simulink model "TeslaCoil"  (R2024a)
settings: Solver=VariableStepAuto  StartTime=0.0  StopTime=10.0  RelTol=1e-3
undefined symbols (not defined in the file): DiscIntNeverNeededParam
libraries: nesl_utility x4, simulink x1
settings Model: Creator=Perij  LastModifiedBy=Perij

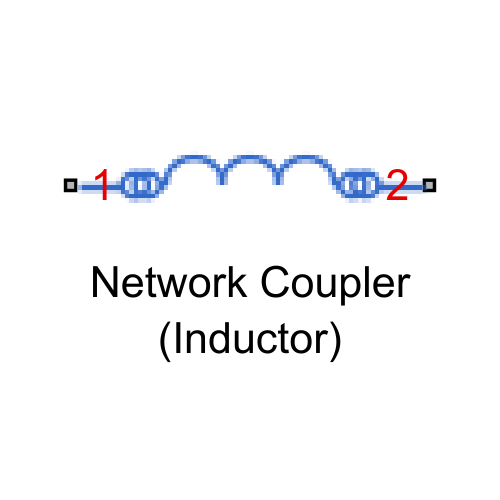
[thumbnail: Simulink's stored preview of the top-level diagram]
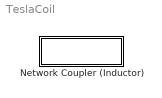
== system TeslaCoil ==
  Network Coupler (Inductor) : Subsystem  mask(Network Coupler (Inductor)){}
      mask init:
      | % Icon
      | key = 'Simscape.NetworkCouplers.Inductor';
      | foundation.internal.couplers.updateIcon(gcb,'inductor.svg',key)
      settings: OpenFcn=open_system(gcbh,'force')
      mask Help: web([docroot '/simscape/ref/networkcouplerinductor.html'])
      mask Display:
      | color('red');
      | port_label('LConn', 1,'1')
      | port_label('RConn', 1,'2')

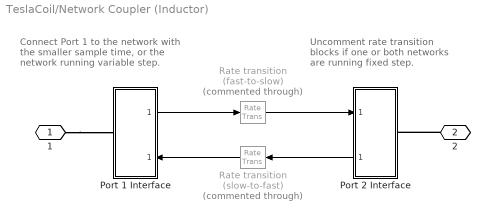
== system TeslaCoil/Network Coupler (Inductor) ==
  note: Connect Port 1 to the network
      | with the smaller sample time, or
      | the network running variable step.
  note: Uncomment rate transition
      | blocks if one or both networks
      | are running fixed step.
  Port 1 Interface : Subsystem  mask(Network Coupler (Inductor) Port 1 Interface){isThreePhase=off, numNodes=1, inductance=1e-3, samplingType=Variable step at ports 1 and 2, h1=0.0002, h2=0.001, predictionDiscreteToContinuous=off, smoothingContinuousToDiscrete=off, predictionSlowToFast=off, smoothingFastToSlow=off, nSmooth=1, tsSmoothing=0.01, rNetwork=0.1, hRecommended=0.001, i0=0}
      mask prompts: isThreePhase "physmod:simscape:couplers:SimscapeNetworkCouplersLib:ElectricalThreePhase_MP"; numNodes "physmod:simscape:couplers:SimscapeNetworkCouplersLib:ElectricalNodeArraySize_MP"; inductance "physmod:simscape:couplers:SimscapeNetworkCouplersLib:InductanceH_MP"; samplingType "physmod:simscape:couplers:SimscapeNetworkCouplersLib:SamplingType_MP"; h1 "physmod:simscape:couplers:SimscapeNetworkCouplersLib:Port1NetworkDiscreteSampleTimes_MP"; h2 "physmod:simscape:couplers:SimscapeNetworkCouplersLib:Port2NetworkDiscreteSampleTimes_MP"; predictionDiscreteToContinuous "physmod:simscape:couplers:SimscapeNetworkCouplersLib:UsePredictionWhenConnectingFixedStepToVariableStep_MP"; smoothingContinuousToDiscrete "physmod:simscape:couplers:SimscapeNetworkCouplersLib:UseSmoothingWhenConnectingVariableStepToFixedStep_MP"; predictionSlowToFast "physmod:simscape:couplers:SimscapeNetworkCouplersLib:UsePredictionWhenConnectingSlowToFastSampleTimes_MP"; smoothingFastToSlow "physmod:simscape:couplers:SimscapeNetworkCouplersLib:UseSmoothingWhenConnectingFastToSlowSampleTimes_MP"; nSmooth "physmod:simscape:couplers:SimscapeNetworkCouplersLib:NumberOfSamplesOverWhichToSmooth_MP"; tsSmoothing "physmod:simscape:couplers:SimscapeNetworkCouplersLib:SmoothingTimeConstants_MP"; rNetwork "physmod:simscape:couplers:SimscapeNetworkCouplersLib:ApproximateConnectedNetworkImpedanceohms_MP"; hRecommended "physmod:simscape:couplers:SimscapeNetworkCouplersLib:RecommendedMaxDiscreteSampleTimes_MP"; i0 "physmod:simscape:couplers:SimscapeNetworkCouplersLib:InitialCurrentA_MP"
      mask help: physmod:simscape:couplers:SimscapeNetworkCouplersLib:NetworkCouplerInductorPort1Interface_MD
      mask init:
      | % Fixed step sample time value check
      | foundation.internal.couplers.checkSampleTimes(gcb,h1,h2);
      | 
      | % Remaining parameter value checks
      | foundation.internal.couplers.electrical.checkParametersInductor(inductance,isThreePhase,numNodes,i0);
      settings: PortSchema="{\"entries\":[{\"content\":{\"sides\":[{\"content\":{\"connectorIds\":[\"LConn1\"]},\"type\":\"ConnectorPlacement.EquallySpacedRectSide\",\"uuid\":\"a6d4a9fd-b5aa-40dc-ab7e-2b646b9b57bc\"},{\"content\":{\"connectorIds\":[\"Out1\",\"In1\"],\"side\":\"RIGHT\"},\"type\":\"ConnectorPlacement.EquallySpacedRectSide\",\"uuid\":\"31bb6273-5b9b-48d0-a1a2-6fbacb979b97\"},{\"content\":{\"connectorIds\":[],\"side\":\"TOP\"},\"type\":\"ConnectorPlacement.EquallySpacedRectSide\",\"uuid\":\"0f7afab2-4481-486c-9ad0-2b42c5b091a4\"}]},\"type\":\"ConnectorPlacement.EquallySpacedConnector\",\"uuid\":\"a98e47aa-cbfd-441a-b14c-c9ea515c056e\"}],\"packageUris\":[\"http://schema.mathworks.com/mf0/Connector/R2020b\"],\"version\":\"1.0\"}"
      mask Help: web([docroot '/simscape/ref/networkcouplerinductor.html'])
      mask Callback isThreePhase: foundation.internal.couplers.electrical.parameterVisibilitiesThreePhase(gcb)
      mask TypeOptions samplingType: physmod:simscape:couplers:SimscapeNetworkCouplersLib:VariableStepAtPorts1And2_PV | physmod:simscape:couplers:SimscapeNetworkCouplersLib:VariableStepAtPort1AndFixedStepAtPort2_PV | physmod:simscape:couplers:SimscapeNetworkCouplersLib:FixedStepBothPortsWithCommonSampleTime_PV | physmod:simscape:couplers:SimscapeNetworkCouplersLib:FixedStepBothPortsWithFasterSamplingAtPort1_PV
      mask Callback samplingType: foundation.internal.couplers.electrical.parameterVisibilities(gcb)
      mask Callback predictionDiscreteToContinuous: foundation.internal.couplers.electrical.parameterVisibilities(gcb)
      mask Callback smoothingContinuousToDiscrete: foundation.internal.couplers.electrical.parameterVisibilities(gcb)
      mask Callback predictionSlowToFast: foundation.internal.couplers.electrical.parameterVisibilities(gcb)
      mask Callback smoothingFastToSlow: foundation.internal.couplers.electrical.parameterVisibilities(gcb)
      mask DialogControl Main Prompt: physmod:simscape:couplers:SimscapeNetworkCouplersLib:tab_Main
      mask DialogControl isThreePhase Prompt: Use three-phase electrical connections
      mask DialogControl numNodes Prompt: Electrical node array size
      mask DialogControl inductance Prompt: Inductance (H)
      mask DialogControl samplingType Prompt: Sampling type
      mask DialogControl h1 Prompt: Port 1 network discrete sample time (s)
      mask DialogControl h2 Prompt: Port 2 network discrete sample time (s)
      mask DialogControl predictionDiscreteToContinuous Prompt: Use prediction when connecting fixed step to variable step
      mask DialogControl smoothingContinuousToDiscrete Prompt: Use smoothing when connecting variable step to fixed step
      mask DialogControl predictionSlowToFast Prompt: Use prediction when connecting slow to fast sample times
      mask DialogControl smoothingFastToSlow Prompt: Use smoothing when connecting fast to slow sample times
      mask DialogControl nSmooth Prompt: Number of samples over which to smooth
      mask DialogControl tsSmoothing Prompt: Smoothing time constant (s)
      mask DialogControl Analysis Prompt: physmod:simscape:couplers:SimscapeNetworkCouplersLib:tab_Analysis
      mask DialogControl connectedNetworkInfo Prompt: physmod:simscape:couplers:SimscapeNetworkCouplersLib:heading_ConnectedNetworkInformation
      mask DialogControl rNetwork Prompt: Approximate connected network resistance (ohms)
      mask DialogControl derivedValues Prompt: physmod:simscape:couplers:SimscapeNetworkCouplersLib:heading_DerivedValues
      mask DialogControl hRecommended Prompt: Recommended max discrete sample time (s)
      mask DialogControl updateRecommendations Prompt: physmod:simscape:couplers:SimscapeNetworkCouplersLib:button_Update
      mask DialogControl updateRecommendations Callback: foundation.internal.couplers.electrical.analysisInductor(gcb);
      mask DialogControl InitialConditions Prompt: physmod:simscape:couplers:SimscapeNetworkCouplersLib:tab_InitialConditions
      mask DialogControl i0 Prompt: Initial current (A)
  Port 2 Interface : Subsystem  mask(Network Coupler (Inductor) Port 2 Interface){isThreePhase=off, numNodes=1}
      mask prompts: isThreePhase "physmod:simscape:couplers:SimscapeNetworkCouplersLib:ElectricalThreePhase_MP"; numNodes "physmod:simscape:couplers:SimscapeNetworkCouplersLib:ElectricalNodeArraySize_MP"
      mask help: physmod:simscape:couplers:SimscapeNetworkCouplersLib:NetworkCouplerInductorPort2Interface_MD
      mask init:
      | % Parameter value checks
      | foundation.internal.couplers.electrical.checkParametersNumNodes(isThreePhase,numNodes);
      settings: PortSchema="{\"entries\":[{\"content\":{\"sides\":[{\"content\":{\"connectorIds\":[\"In1\",\"Out1\"]},\"type\":\"ConnectorPlacement.EquallySpacedRectSide\",\"uuid\":\"5a4c1550-e77d-42df-bf3e-b81963920de7\"},{\"content\":{\"connectorIds\":[\"RConn1\"],\"side\":\"RIGHT\"},\"type\":\"ConnectorPlacement.EquallySpacedRectSide\",\"uuid\":\"3fd730f7-5937-4563-a365-595aaae9027b\"},{\"content\":{\"connectorIds\":[],\"side\":\"TOP\"},\"type\":\"ConnectorPlacement.EquallySpacedRectSide\",\"uuid\":\"c16e04e4-26e8-4fd6-98d3-59adbef44c0d\"}]},\"type\":\"ConnectorPlacement.EquallySpacedConnector\",\"uuid\":\"5588d8d0-d459-45fe-a303-1ca6654e99d0\"}],\"packageUris\":[\"http://schema.mathworks.com/mf0/Connector/R2020b\"],\"version\":\"1.0\"}"
      mask Help: web([docroot '/simscape/ref/networkcouplerinductor.html'])
      mask Callback isThreePhase: foundation.internal.couplers.electrical.parameterVisibilitiesThreePhase(gcb)
      mask DialogControl isThreePhase Prompt: Use three-phase electrical connections
      mask DialogControl numNodes Prompt: Electrical node array size
  Rate transition (fast-to-slow) : RateTransition  Commented=through  Integrity=off
  Rate transition (slow-to-fast) : RateTransition  Commented=through  Integrity=off
  1 : PMIOPort  Side=Left
  2 : PMIOPort  Port=2  Side=Right
  wires:
  Rate transition (fast-to-slow)/1 -> Port 2 Interface/1(current)
  Rate transition (slow-to-fast)/1 -> Port 1 Interface/1(voltage)
  Port 2 Interface/1(voltage) -> Rate transition (slow-to-fast)/1
  Port 1 Interface/1(current) -> Rate transition (fast-to-slow)/1
  connections:
  1/RConn1 -- Port 1 Interface/LConn1
  2/RConn1 -- Port 2 Interface/RConn1

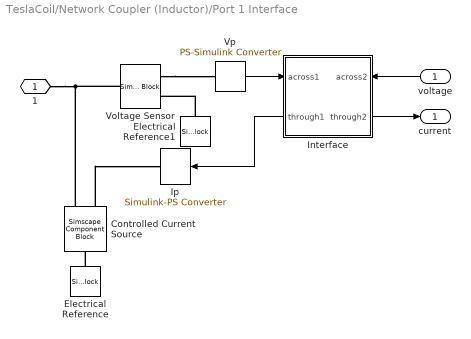
== system TeslaCoil/Network Coupler (Inductor)/Port 1 Interface ==
  voltage : Inport
  Controlled Current Source : SimscapeComponentBlock  SourceFile=foundation.internal.couplers.electrical.currentSource  ComponentPath=foundation.internal.couplers.electrical.currentSource  ComponentVariants="[\"foundation.internal.couplers.electrical.currentSource\"]"  ComponentVariantNames="[\"currentSource\"]"  ClassName=currentSource  SchemaVersion=1  threePhase=false  numNodes=numNodes
      settings: CopyFcn=simscape.engine.sli.internal.componentblockcallback(gcbh,'COPY')  PreCopyFcn=simscape.engine.sli.internal.componentblockcallback(gcbh,'PRECOPY')  PreDeleteFcn=simscape.engine.sli.internal.componentblockcallback(gcbh,'PREDELETE')  InternalSimscapePortConfiguration="{\"Bottom\":[],\"Left\":[{\"id\":\"head\",\"label\":\"\",\"type\":\"foundation.electrical.electrical\"}],\"Right\":[{\"id\":\"iT\",\"label\":\"\",\"type\":\"input\"},{\"id\":\"tail\",\"label\":\"\",\"type\":\"foundation.electrical.electrical\"}],\"Top\":[]}"
      mask Type: Controlled Current Source
  Electrical Reference : SimscapeComponentBlock  SourceFile=foundation.internal.couplers.electrical.reference  ComponentPath=foundation.internal.couplers.electrical.reference  ComponentVariants="[\"foundation.internal.couplers.electrical.reference\"]"  ComponentVariantNames="[\"reference\"]"  ClassName=reference  SchemaVersion=1  threePhase=false  numNodes=numNodes
      settings: CopyFcn=simscape.engine.sli.internal.componentblockcallback(gcbh,'COPY')  PreCopyFcn=simscape.engine.sli.internal.componentblockcallback(gcbh,'PRECOPY')  PreDeleteFcn=simscape.engine.sli.internal.componentblockcallback(gcbh,'PREDELETE')  InternalSimscapePortConfiguration="{\"Bottom\":[],\"Left\":[{\"id\":\"p\",\"label\":\"\",\"type\":\"foundation.electrical.electrical\"}],\"Right\":[],\"Top\":[]}"
      mask Type: Electrical Reference
  Electrical Reference1 : SimscapeComponentBlock  SourceFile=foundation.internal.couplers.electrical.reference  ComponentPath=foundation.internal.couplers.electrical.reference  ComponentVariants="[\"foundation.internal.couplers.electrical.reference\"]"  ComponentVariantNames="[\"reference\"]"  ClassName=reference  SchemaVersion=1  threePhase=false  numNodes=numNodes
      settings: CopyFcn=simscape.engine.sli.internal.componentblockcallback(gcbh,'COPY')  PreCopyFcn=simscape.engine.sli.internal.componentblockcallback(gcbh,'PRECOPY')  PreDeleteFcn=simscape.engine.sli.internal.componentblockcallback(gcbh,'PREDELETE')  InternalSimscapePortConfiguration="{\"Bottom\":[],\"Left\":[{\"id\":\"p\",\"label\":\"\",\"type\":\"foundation.electrical.electrical\"}],\"Right\":[],\"Top\":[]}"
      mask Type: Electrical Reference
  Interface : Subsystem  Variant=on  VariantControlMode=label  VariantControl=Variant1  LabelModeActiveChoice=Continuous
      settings: PortSchema="{\"entries\":[{\"content\":{\"sides\":[{\"content\":{\"connectorIds\":[\"In1\",\"Out2\"]},\"type\":\"ConnectorPlacement.EquallySpacedRectSide\",\"uuid\":\"aa56821c-7799-44e3-b228-553c5b43a68d\"},{\"content\":{\"connectorIds\":[\"In2\",\"Out1\"],\"side\":\"RIGHT\"},\"type\":\"ConnectorPlacement.EquallySpacedRectSide\",\"uuid\":\"8658dee5-55e2-4f33-bdec-e6600ce27fc1\"},{\"content\":{\"connectorIds\":[],\"side\":\"TOP\"},\"type\":\"ConnectorPlacement.EquallySpacedRectSide\",\"uuid\":\"2effe9c6-8e61-4f0c-a39b-329d9ffc707d\"}]},\"type\":\"ConnectorPlacement.EquallySpacedConnector\",\"uuid\":\"c8fc8444-dfc7-49a5-9550-b957635f7d8f\"}],\"packageUris\":[\"http://schema.mathworks.com/mf0/Connector/R2020b\"],\"version\":\"1.0\"}"
  Ip : nesl_utility/Simulink-PS Converter  PhysicalDomain=network_engine_domain  SubClassName=ps_input  LeftPortType=input  RightPortType=output  PseudoPeriodic=off  Frequencies=[]  NoiseDistribution=none  NoiseParameters=[]  Unit=A  AffineConversion=off  FilteringAndDerivatives=zero  SimscapeFilterOrder=1  InputFilterTimeConstant=0.001  UdotUserProvided=1
  Voltage Sensor : SimscapeComponentBlock  SourceFile=foundation.internal.couplers.electrical.voltageSensor  ComponentPath=foundation.internal.couplers.electrical.voltageSensor  ComponentVariants="[\"foundation.internal.couplers.electrical.voltageSensor\"]"  ComponentVariantNames="[\"voltageSensor\"]"  ClassName=voltageSensor  SchemaVersion=1  threePhase=false  numNodes=numNodes
      settings: CopyFcn=simscape.engine.sli.internal.componentblockcallback(gcbh,'COPY')  PreCopyFcn=simscape.engine.sli.internal.componentblockcallback(gcbh,'PRECOPY')  PreDeleteFcn=simscape.engine.sli.internal.componentblockcallback(gcbh,'PREDELETE')  InternalSimscapePortConfiguration="{\"Bottom\":[],\"Left\":[{\"id\":\"p\",\"label\":\"+\",\"type\":\"foundation.electrical.electrical\"}],\"Right\":[{\"id\":\"V\",\"label\":\"V\",\"type\":\"output\"},{\"id\":\"n\",\"label\":\"-\",\"type\":\"foundation.electrical.electrical\"}],\"Top\":[]}"
      mask Type: Voltage Sensor
  Vp : nesl_utility/PS-Simulink Converter  PhysicalDomain=network_engine_domain  SubClassName=ps_output  LeftPortType=input  RightPortType=output  PseudoPeriodic=off  Frequencies=[]  VectorFormat=1-D array  Unit=V  AffineConversion=off
  1 : PMIOPort  Side=Left
  current : Outport
  wires:
  voltage/1 -> Interface/2(across2)
  Interface/2(through1) -> Ip/1
  Vp/1 -> Interface/1(across1)
  Interface/1(through2) -> current/1
  connections:
  Controlled Current Source/RConn1 -- Ip/RConn1
  Electrical Reference/LConn1 -- Controlled Current Source/LConn1
  Electrical Reference1/LConn1 -- Voltage Sensor/RConn2
  Controlled Current Source/RConn2 -- Voltage Sensor/LConn1 -- 1/RConn1
  Voltage Sensor/RConn1 -- Vp/LConn1

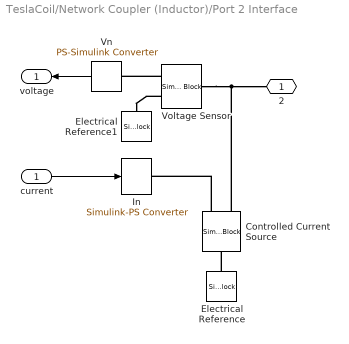
== system TeslaCoil/Network Coupler (Inductor)/Port 2 Interface ==
  current : Inport
  Controlled Current Source : SimscapeComponentBlock  SourceFile=foundation.internal.couplers.electrical.currentSource  ComponentPath=foundation.internal.couplers.electrical.currentSource  ComponentVariants="[\"foundation.internal.couplers.electrical.currentSource\"]"  ComponentVariantNames="[\"currentSource\"]"  ClassName=currentSource  SchemaVersion=1  threePhase=false  numNodes=numNodes
      settings: CopyFcn=simscape.engine.sli.internal.componentblockcallback(gcbh,'COPY')  PreCopyFcn=simscape.engine.sli.internal.componentblockcallback(gcbh,'PRECOPY')  PreDeleteFcn=simscape.engine.sli.internal.componentblockcallback(gcbh,'PREDELETE')  InternalSimscapePortConfiguration="{\"Bottom\":[],\"Left\":[{\"id\":\"head\",\"label\":\"\",\"type\":\"foundation.electrical.electrical\"}],\"Right\":[{\"id\":\"iT\",\"label\":\"\",\"type\":\"input\"},{\"id\":\"tail\",\"label\":\"\",\"type\":\"foundation.electrical.electrical\"}],\"Top\":[]}"
      mask Type: Controlled Current Source
  Electrical Reference : SimscapeComponentBlock  SourceFile=foundation.internal.couplers.electrical.reference  ComponentPath=foundation.internal.couplers.electrical.reference  ComponentVariants="[\"foundation.internal.couplers.electrical.reference\"]"  ComponentVariantNames="[\"reference\"]"  ClassName=reference  SchemaVersion=1  threePhase=false  numNodes=numNodes
      settings: CopyFcn=simscape.engine.sli.internal.componentblockcallback(gcbh,'COPY')  PreCopyFcn=simscape.engine.sli.internal.componentblockcallback(gcbh,'PRECOPY')  PreDeleteFcn=simscape.engine.sli.internal.componentblockcallback(gcbh,'PREDELETE')  InternalSimscapePortConfiguration="{\"Bottom\":[],\"Left\":[{\"id\":\"p\",\"label\":\"\",\"type\":\"foundation.electrical.electrical\"}],\"Right\":[],\"Top\":[]}"
      mask Type: Electrical Reference
  Electrical Reference1 : SimscapeComponentBlock  SourceFile=foundation.internal.couplers.electrical.reference  ComponentPath=foundation.internal.couplers.electrical.reference  ComponentVariants="[\"foundation.internal.couplers.electrical.reference\"]"  ComponentVariantNames="[\"reference\"]"  ClassName=reference  SchemaVersion=1  threePhase=false  numNodes=numNodes
      settings: CopyFcn=simscape.engine.sli.internal.componentblockcallback(gcbh,'COPY')  PreCopyFcn=simscape.engine.sli.internal.componentblockcallback(gcbh,'PRECOPY')  PreDeleteFcn=simscape.engine.sli.internal.componentblockcallback(gcbh,'PREDELETE')  InternalSimscapePortConfiguration="{\"Bottom\":[],\"Left\":[{\"id\":\"p\",\"label\":\"\",\"type\":\"foundation.electrical.electrical\"}],\"Right\":[],\"Top\":[]}"
      mask Type: Electrical Reference
  In : nesl_utility/Simulink-PS Converter  PhysicalDomain=network_engine_domain  SubClassName=ps_input  LeftPortType=input  RightPortType=output  PseudoPeriodic=off  Frequencies=[]  NoiseDistribution=none  NoiseParameters=[]  Unit=A  AffineConversion=off  FilteringAndDerivatives=zero  SimscapeFilterOrder=1  InputFilterTimeConstant=0.001  UdotUserProvided=1
  Vn : nesl_utility/PS-Simulink Converter  PhysicalDomain=network_engine_domain  SubClassName=ps_output  LeftPortType=input  RightPortType=output  PseudoPeriodic=off  Frequencies=[]  VectorFormat=1-D array  Unit=V  AffineConversion=off
  Voltage Sensor : SimscapeComponentBlock  SourceFile=foundation.internal.couplers.electrical.voltageSensor  ComponentPath=foundation.internal.couplers.electrical.voltageSensor  ComponentVariants="[\"foundation.internal.couplers.electrical.voltageSensor\"]"  ComponentVariantNames="[\"voltageSensor\"]"  ClassName=voltageSensor  SchemaVersion=1  threePhase=false  numNodes=numNodes
      settings: CopyFcn=simscape.engine.sli.internal.componentblockcallback(gcbh,'COPY')  PreCopyFcn=simscape.engine.sli.internal.componentblockcallback(gcbh,'PRECOPY')  PreDeleteFcn=simscape.engine.sli.internal.componentblockcallback(gcbh,'PREDELETE')  InternalSimscapePortConfiguration="{\"Bottom\":[],\"Left\":[{\"id\":\"p\",\"label\":\"+\",\"type\":\"foundation.electrical.electrical\"}],\"Right\":[{\"id\":\"V\",\"label\":\"V\",\"type\":\"output\"},{\"id\":\"n\",\"label\":\"-\",\"type\":\"foundation.electrical.electrical\"}],\"Top\":[]}"
      mask Type: Voltage Sensor
  2 : PMIOPort  Side=Right
  voltage : Outport
  wires:
  current/1 -> In/1
  Vn/1 -> voltage/1
  connections:
  Controlled Current Source/RConn1 -- In/RConn1
  Electrical Reference/LConn1 -- Controlled Current Source/LConn1
  Voltage Sensor/RConn2 -- Electrical Reference1/LConn1
  Voltage Sensor/RConn1 -- Vn/LConn1
  Controlled Current Source/RConn2 -- Voltage Sensor/LConn1 -- 2/RConn1

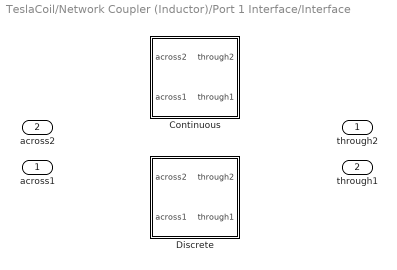
== system TeslaCoil/Network Coupler (Inductor)/Port 1 Interface/Interface ==
  across1 : Inport
  across2 : Inport  Port=2
  Continuous : Subsystem  VariantControl=Continuous
  Discrete : Subsystem  VariantControl=Discrete
  through2 : Outport
  through1 : Outport  Port=2

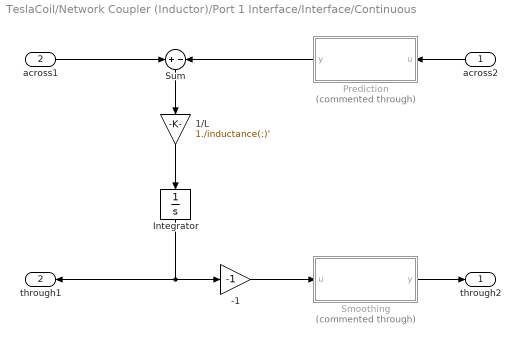
== system TeslaCoil/Network Coupler (Inductor)/Port 1 Interface/Interface/Continuous ==
  across2 : Inport
  across1 : Inport  Port=2
  -1 : Gain  Gain=-1  SaturateOnIntegerOverflow=on  OutDataTypeStr=Inherit: Same as input  ParamDataTypeStr=Inherit: Same as input
  1/L : Gain  Gain=1./inductance(:)'  SaturateOnIntegerOverflow=on  OutDataTypeStr=Inherit: Same as input  ParamDataTypeStr=Inherit: Same as input
  Integrator : Integrator  InitialCondition=i0
  Prediction : Subsystem  Commented=through  mask(Prediction (discrete->continuous)){h2=h2}
      mask prompts: h2 "physmod:simscape:couplers:SimscapeNetworkCouplersLib:PortUDiscreteSampleTimes_MP"
      mask help: physmod:simscape:couplers:SimscapeNetworkCouplersLib:Predictiondiscretecontinuous_MD
      mask DialogControl h2 Prompt: Port u discrete sample time (s)
  Smoothing : Subsystem  Commented=through  mask(Smoothing (continuous->discrete)){tsSmoothing=tsSmoothing, smoothing0=i0}
      mask prompts: tsSmoothing "physmod:simscape:couplers:SimscapeNetworkCouplersLib:SmoothingTimeConstants_MP"; smoothing0 "physmod:simscape:couplers:SimscapeNetworkCouplersLib:InitialOutput_MP"
      mask help: physmod:simscape:couplers:SimscapeNetworkCouplersLib:Smoothingcontinuousdiscrete_MD
      mask DialogControl tsSmoothing Prompt: Smoothing time constant (s)
      mask DialogControl smoothing0 Prompt: Initial output
  Sum : Sum  Inputs=+-  InputSameDT=on  SaturateOnIntegerOverflow=on  OutDataTypeStr=Inherit: Same as first input
  through2 : Outport
  through1 : Outport  Port=2
  wires:
  Integrator/1 -> -1/1, through1/1
  Sum/1 -> 1/L/1
  -1/1 -> Smoothing/1(u)
  1/L/1 -> Integrator/1
  across2/1 -> Prediction/1(u)
  across1/1 -> Sum/1
  Prediction/1(y) -> Sum/2
  Smoothing/1(y) -> through2/1

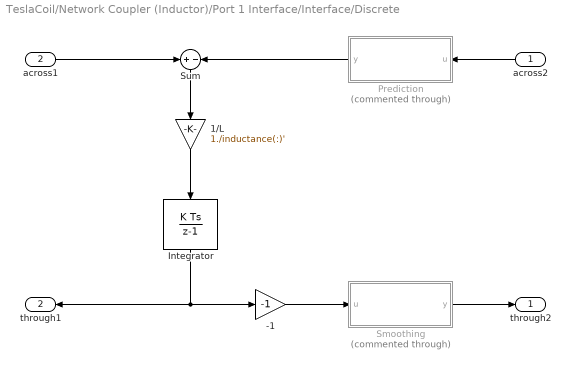
== system TeslaCoil/Network Coupler (Inductor)/Port 1 Interface/Interface/Discrete ==
  across2 : Inport
  across1 : Inport  Port=2
  -1 : Gain  Gain=-1  SaturateOnIntegerOverflow=on  OutDataTypeStr=Inherit: Same as input  ParamDataTypeStr=Inherit: Same as input
  1/L : Gain  Gain=1./inductance(:)'  SaturateOnIntegerOverflow=on  OutDataTypeStr=Inherit: Same as input  ParamDataTypeStr=Inherit: Same as input
  Integrator : DiscreteIntegrator  InitialCondition=i0  SampleTime=h1  ICPrevOutput=DiscIntNeverNeededParam  ICPrevScaledInput=DiscIntNeverNeededParam
  Prediction : Subsystem  Commented=through  mask(Prediction (slow->fast)){h2=h2, h1=h1}
      mask prompts: h2 "physmod:simscape:couplers:SimscapeNetworkCouplersLib:PortUDiscreteSampleTimes_MP"; h1 "physmod:simscape:couplers:SimscapeNetworkCouplersLib:PortYDiscreteSampleTimes_MP"
      mask help: physmod:simscape:couplers:SimscapeNetworkCouplersLib:Predictionslowfast_MD
      mask DialogControl h2 Prompt: Port u discrete sample time (s)
      mask DialogControl h1 Prompt: Port y discrete sample time (s)
  Smoothing : Subsystem  Commented=through  mask(Smoothing (fast->slow)){nSmooth=nSmooth, h1=h1, smoothing0=i0}
      mask prompts: nSmooth "physmod:simscape:couplers:SimscapeNetworkCouplersLib:NumberOfSamplesOverWhichToSmooth_MP"; h1 "physmod:simscape:couplers:SimscapeNetworkCouplersLib:PortUDiscreteSampleTimes_MP"; smoothing0 "physmod:simscape:couplers:SimscapeNetworkCouplersLib:InitialOutput_MP"
      mask help: physmod:simscape:couplers:SimscapeNetworkCouplersLib:Smoothingfastslow_MD
      mask DialogControl nSmooth Prompt: Number of samples over which to smooth
      mask DialogControl h1 Prompt: Port u discrete sample time (s)
      mask DialogControl smoothing0 Prompt: Initial output
  Sum : Sum  Inputs=+-  InputSameDT=on  SaturateOnIntegerOverflow=on  OutDataTypeStr=Inherit: Same as first input
  through2 : Outport
  through1 : Outport  Port=2
  wires:
  Integrator/1 -> -1/1, through1/1
  Sum/1 -> 1/L/1
  -1/1 -> Smoothing/1(u)
  across1/1 -> Sum/1
  across2/1 -> Prediction/1(u)
  1/L/1 -> Integrator/1
  Prediction/1(y) -> Sum/2
  Smoothing/1(y) -> through2/1

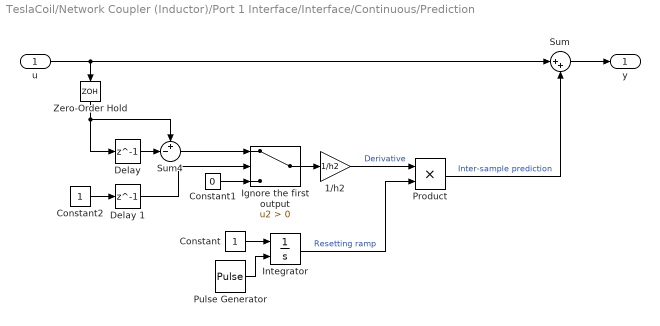
== system TeslaCoil/Network Coupler (Inductor)/Port 1 Interface/Interface/Continuous/Prediction ==
  u : Inport
  1/h2 : Gain  Gain=1/h2
  Constant : Constant  SampleTime=h2
  Constant1 : Constant  Value=0  SampleTime=h2
  Constant2 : Constant  SampleTime=h2
  "Delay " : Delay  DelayLength=1  SampleTime=h2
  Delay 1 : Delay  DelayLength=1  SampleTime=h2
  Ignore the first output : Switch  Criteria=u2 > Threshold  SaturateOnIntegerOverflow=off  InputSameDT=off
  Integrator : Integrator  ExternalReset=either  LimitOutput=on  UpperSaturationLimit=1  LowerSaturationLimit=0
  Product : Product
  Pulse Generator : DiscretePulseGenerator  SampleTime=h2
  Sum : Sum  Inputs=|++
  Sum4 : Sum  Inputs=+-|
  Zero-Order Hold : ZeroOrderHold  SampleTime=h2
  y : Outport
  wires:
  Constant2/1 -> Delay 1/1
  Delay 1/1 -> Ignore the first output/2
  Constant1/1 -> Ignore the first output/3
  Sum4/1 -> Ignore the first output/1
  Ignore the first output/1 -> 1/h2/1
  Pulse Generator/1 -> Integrator/2
  Constant/1 -> Integrator/1
  Integrator/1 -> Product/2  "Resetting ramp"
  Sum/1 -> y/1
  1/h2/1 -> Product/1  "Derivative"
  "Delay "/1 -> Sum4/2
  u/1 -> Zero-Order Hold/1, Sum/1
  Zero-Order Hold/1 -> "Delay "/1, Sum4/1
  Product/1 -> Sum/2  "Inter-sample prediction"

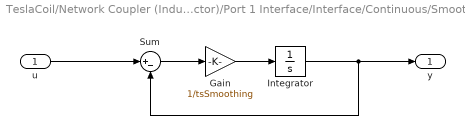
== system TeslaCoil/Network Coupler (Inductor)/Port 1 Interface/Interface/Continuous/Smoothing ==
  u : Inport
  Gain : Gain  Gain=1/tsSmoothing
  Integrator : Integrator  InitialCondition=smoothing0
  Sum : Sum  Inputs=|+-
  y : Outport
  wires:
  Sum/1 -> Gain/1
  Gain/1 -> Integrator/1
  Integrator/1 -> y/1, Sum/2
  u/1 -> Sum/1

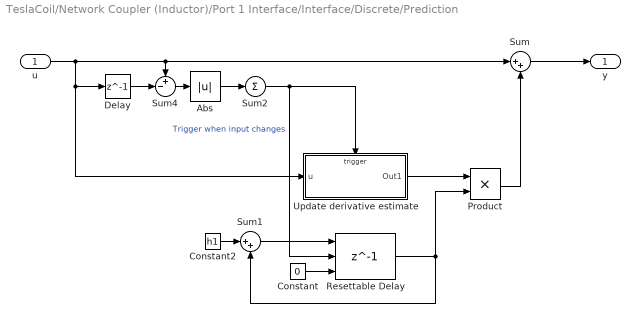
== system TeslaCoil/Network Coupler (Inductor)/Port 1 Interface/Interface/Discrete/Prediction ==
  u : Inport
  Abs : Abs  SaturateOnIntegerOverflow=off
  Constant : Constant  Value=0  SampleTime=h1
  Constant2 : Constant  Value=h1  SampleTime=h1
  "Delay " : Delay  DelayLength=1  SampleTime=h1
  Product : Product
  Resettable Delay : Delay  DelayLength=1  InitialConditionSource=Input port  ExternalReset=Either  SampleTime=h1
      settings: InputPortMap=u0,r5,p4
  Sum : Sum  Inputs=|++
  Sum1 : Sum  Inputs=|++
  Sum2 : Sum  Inputs=+
  Sum4 : Sum  Inputs=+-|
  Update derivative estimate : Subsystem  TreatAsAtomicUnit=on
  y : Outport
  wires:
  Constant/1 -> Resettable Delay/3
  Constant2/1 -> Sum1/1
  Resettable Delay/1 -> Sum1/2, Product/2
  Sum4/1 -> Abs/1
  u/1 -> Sum4/1, Sum/1, "Delay "/1, Update derivative estimate/1(u)
  Update derivative estimate/1(Out1) -> Product/1
  Product/1 -> Sum/2
  "Delay "/1 -> Sum4/2
  Sum/1 -> y/1
  Sum1/1 -> Resettable Delay/1
  Sum2/1 -> Update derivative estimate/Trigger, Resettable Delay/2  "Trigger when input changes"
  Abs/1 -> Sum2/1

== system TeslaCoil/Network Coupler (Inductor)/Port 1 Interface/Interface/Discrete/Smoothing ==
  u : Inport
  For Each Subsystem : Subsystem  TreatAsAtomicUnit=on
  y : Outport
  wires:
  For Each Subsystem/1(y) -> y/1
  u/1 -> For Each Subsystem/1(u)

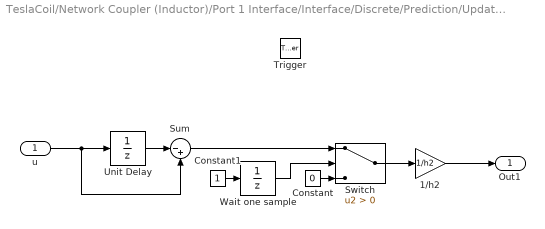
== system TeslaCoil/Network Coupler (Inductor)/Port 1 Interface/Interface/Discrete/Prediction/Update derivative estimate ==
  u : Inport
  Trigger : TriggerPort  TriggerType=either  VariantControl=(inherit)
  1/h2 : Gain  Gain=1/h2
  Constant : Constant  Value=0  SampleTime=-1
  Constant1 : Constant  SampleTime=-1
  Sum : Sum  Inputs=|-+
  Switch : Switch  Criteria=u2 > Threshold  SaturateOnIntegerOverflow=off  InputSameDT=off
  Unit Delay : UnitDelay  SampleTime=-1  HasFrameUpgradeWarning=on
  Wait one sample : UnitDelay  SampleTime=-1  HasFrameUpgradeWarning=on
  Out1 : Outport
  wires:
  Constant1/1 -> Wait one sample/1
  Wait one sample/1 -> Switch/2
  Constant/1 -> Switch/3
  Sum/1 -> Switch/1
  Switch/1 -> 1/h2/1
  1/h2/1 -> Out1/1
  u/1 -> Sum/2, Unit Delay/1
  Unit Delay/1 -> Sum/1

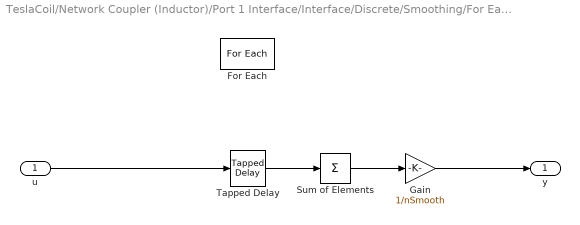
== system TeslaCoil/Network Coupler (Inductor)/Port 1 Interface/Interface/Discrete/Smoothing/For Each Subsystem ==
  u : Inport  Partition=on  PartitionDimension=1  PartitionWidth=1  PartitionOffset=0
  For Each : ForEach  DisableCoverage=on
  Gain : Gain  Gain=1/nSmooth
  Sum of Elements : Sum  Inputs=+
  Tapped Delay : simulink/Discrete/Tapped Delay  vinit=mean(smoothing0)  samptime=h1  NumDelays=nSmooth  DelayOrder=Oldest  includeCurrent=off
      settings: LibrarySourceBlock=|
      | SimscapeNetworkCouplersLib/Fundamental Components/Smoothing (fast->slow)/For Each
      | Subsystem/Tapped Delay
  y : Outport  ConcatenationDimension=1
  wires:
  Gain/1 -> y/1
  Tapped Delay/1 -> Sum of Elements/1
  Sum of Elements/1 -> Gain/1
  u/1 -> Tapped Delay/1
